simulink model "modules"  (R2017a)
settings: Solver=ode4  StartTime=0.0  StopTime=time_stop  FixedStep=time_step  RelTol=1e-3
values from neighbouring files (symbols this model uses):
  psi = state(3)    [PSVobstacleShip_class.m]    (also in PSVvessel_class.m = obj.eta(3); PsiReferenceModel_class.m = obj.desired_psi_vector; SBMPC_PSVvessel_class.m = obj.eta(3))
undefined symbols (not defined in the file or in its folder): beta, Delta_guidance, Delta_matrix, eta_initial, initial_desired_psi_vector, initial_desired_u_vector, initial_next_waypoint_indexes, initial_obstacle_ship_states, initial_obstacle_ship_states_dot, initial_reference_psi_vector, initial_reference_u_vector, initial_SBMPC_desired_psi_vector, initial_SBMPC_desired_u_vector, initial_SBMPC_next_waypoint_indexes, initial_SBMPC_obstacle_ship_states, initial_SBMPC_obstacle_ship_states_dot, initial_SBMPC_reference_psi_vector, initial_SBMPC_reference_u_vector, initial_SBMPC_x_d_psi_matrix, initial_SBMPC_x_d_u_matrix, initial_state, initial_x_d_psi_matrix, initial_x_d_u_matrix, K_sway, K_yaw, Kp_feedback_linearization, kp_heading, Nmax, nu_initial, num_obs_ship_waypoints, num_prediction_time_steps, number_of_control_behaviors, number_of_obstacle_ships, number_of_SBMPC_obstacle_ships, obs_speed_between_waypoints, obstacle_waypoint_matrix, Omega_matrix, own_ship_reference_psi_init, own_ship_reference_speed, Psi_init, radius_of_acceptance, SBMPC_obs_speed_between_waypoints, SBMPC_obstacle_waypoint_matrix, seconds_between_prediction, state_vector_init, T, T_k_surge, T_k_sway, T_k_yaw, T_s, T_waypoints, time_step, tsamp, U, U_init, V_init, waypoints_obstacle_ships, waypoints_own_ship, Xmax, Ymax
(part 4 of 5)

== matlab function modules/SBMPC obstacle ships/SBMPC using intentions /Calculate control behaviors/Compute hazard ==
  settings: updateMethod=DISCRETE  sampleTime=time_step
  data: obstacle_ships_u_input input size=[1 + number_of_obstacle_ships, num_prediction_time_steps]; obstacle_ships_v_input input size=[1 + number_of_obstacle_ships, num_prediction_time_steps]; obstacle_ships_psi_input input size=[1 + number_of_obstacle_ships, num_prediction_time_steps]; t_0 input; SBMPC_obstacles_own_ship_x_predicted input size=[number_of_SBMPC_obstacle_ships, num_prediction_time_steps, number_of_control_behaviors]; SBMPC_obstacles_own_ship_y_predicted input size=[number_of_SBMPC_obstacle_ships, num_prediction_time_steps, number_of_control_behaviors]; SBMPC_obstacles_own_ship_u_predicted input size=[number_of_SBMPC_obstacle_ships, num_prediction_time_steps, number_of_control_behaviors]; SBMPC_obstacles_own_ship_v_predicted input size=[number_of_SBMPC_obstacle_ships, num_prediction_time_steps, number_of_control_behaviors]; SBMPC_obstacles_own_ship_heading_predicted input size=[number_of_SBMPC_obstacle_ships, num_prediction_time_steps, number_of_control_behaviors]; CLOSE output size=[number_of_SBMPC_obstacle_ships, number_of_control_behaviors, total_number_of_obstacle_ships, num_prediction_time_steps]; d_0 output size=[number_of_SBMPC_obstacle_ships, number_of_control_behaviors, total_number_of_obstacle_ships, num_prediction_time_steps]; obstacle_ships_x_predicted_input input size=[1 + number_of_obstacle_ships, num_prediction_time_steps]; obstacle_ships_y_predicted_input input size=[1 + number_of_obstacle_ships, num_prediction_time_steps]; OVERTAKEN output size=[number_of_SBMPC_obstacle_ships, number_of_control_behaviors, total_number_of_obstacle_ships, num_prediction_time_steps]; STARBOARD output size=[number_of_SBMPC_obstacle_ships, number_of_control_behaviors, total_number_of_obstacle_ships, num_prediction_time_steps]; chosen_HEAD_ON_out output; CROSSED output size=[number_of_SBMPC_obstacle_ships, number_of_control_behaviors, total_number_of_obstacle_ships, num_prediction_time_steps]; mu output size=[number_of_SBMPC_obstacle_ships, number_of_control_behaviors, total_number_of_obstacle_ships, num_prediction_time_steps]; num_prediction_time_steps parameter; heading_angle_offset_commands parameter; propulsion_commands parameter; total_number_of_obstacle_ships parameter; seconds_between_prediction parameter; d_cl parameter; phi_head_on parameter; phi_crossed parameter; phi_overtaken parameter; phi_ahead parameter; K_coll parameter; C output size=[number_of_SBMPC_obstacle_ships, number_of_control_behaviors, total_number_of_obstacle_ships, num_prediction_time_steps]; R output size=[number_of_SBMPC_obstacle_ships, number_of_control_behaviors, total_number_of_obstacle_ships, num_prediction_time_steps]; q parameter; p parameter; d_safe parameter; k_boundary parameter; k_circle parameter; k_Pr parameter; k_psi_port parameter; k_psi_starboard parameter; Delta_Pr parameter; vessel_length parameter; circle_obstacle_parameters parameter; boundary_obstacles_parameters parameter; k_Delta_psi_port parameter; k_Delta_psi_starboard parameter; kappa parameter; f output size=[number_of_SBMPC_obstacle_ships,number_of_control_behaviors]; g output size=[number_of_SBMPC_obstacle_ships,number_of_control_behaviors]; hazard output size=[number_of_SBMPC_obstacle_ships,number_of_control_behaviors]; rad2deg parameter; num_boundary_obstacles parameter; num_circle_obstacles parameter; chosen_C_out output; chosen_FC_out output; chosen_R_out output; chosen_scaled_mu_out output; T_s parameter; chosen_Pr_out output; chosen_psi_ca_out output; C_worst output; R_worst output; scaled_mu_worst output; Pr_worst output; psi_ca_worst output; f_worst_out output; g_worst_out output; smallest_hazard_out output; largest_hazard_out output; f_out output; g_out output; r parameter; circle_safety_margin parameter; p_boundary parameter; p_circle parameter; q_circle parameter; q_boundary parameter; boundary_margin parameter; number_of_control_behaviors parameter; chosen_scenario_index_out output; number_of_SBMPC_obstacle_ships parameter; chosen_scenario_index_out_init parameter; data_out_init parameter; number_of_obstacle_ships parameter; L_FC parameter; k_FC parameter; L_C parameter
function [CLOSE, d_0, OVERTAKEN, STARBOARD, chosen_HEAD_ON_out, CROSSED,mu, C, R, f, g, hazard, chosen_C_out, chosen_FC_out, chosen_R_out, chosen_scaled_mu_out, chosen_Pr_out, chosen_psi_ca_out, C_worst, R_worst, scaled_mu_worst, Pr_worst, psi_ca_worst, f_worst_out, g_worst_out, smallest_hazard_out, largest_hazard_out, f_out, g_out, chosen_scenario_index_out]                         = computeTotalHazard(obstacle_ships_u_input, obstacle_ships_v_input, obstacle_ships_psi_input, t_0,SBMPC_obstacles_own_ship_x_predicted, SBMPC_obstacles_own_ship_y_predicted,SBMPC_obstacles_own_ship_u_predicted,SBMPC_obstacles_own_ship_v_predicted, SBMPC_obstacles_own_ship_heading_predicted, obstacle_ships_x_predicted_input, obstacle_ships_y_predicted_input, num_prediction_time_steps, heading_angle_offset_commands, propulsion_commands, total_number_of_obstacle_ships, seconds_between_prediction, d_cl,phi_head_on, phi_crossed, phi_overtaken,phi_ahead,K_coll, q, p, d_safe,k_boundary, k_circle, k_Pr, k_psi_port, k_psi_starboard, Delta_Pr, vessel_length, circle_obstacle_parameters, boundary_obstacles_parameters, k_Delta_psi_port, k_Delta_psi_starboard,kappa, rad2deg, num_boundary_obstacles, num_circle_obstacles, T_s, r, circle_safety_margin, p_boundary, p_circle, q_circle, q_boundary, boundary_margin, number_of_control_behaviors, number_of_SBMPC_obstacle_ships, chosen_scenario_index_out_init, data_out_init, number_of_obstacle_ships, L_FC, k_FC, L_C)     
    
    persistent chosen_C;
    persistent chosen_scenario_index;
    persistent chosen_R;
    persistent chosen_scaled_mu;
    persistent chosen_HEAD_ON;
    persistent chosen_FC;
    persistent chosen_Pr;
    persistent chosen_psi_ca;
    persistent chosen_Pr_worst;
    persistent chosen_psi_ca_worst;
    persistent f_worst;
    persistent g_worst;
    persistent f_chosen;
    persistent g_chosen;
    persistent smallest_hazard;
    persistent largest_hazard;
    persistent scenario_index_with_min_hazard;
    persistent scenario_index_with_max_hazard;
    
    if (isempty(chosen_C))
        chosen_C              = zeros(number_of_SBMPC_obstacle_ships,number_of_control_behaviors);%chosen_C_init;
        chosen_scenario_index = ones(1,number_of_SBMPC_obstacle_ships)*7;
        chosen_R              = zeros(number_of_SBMPC_obstacle_ships,number_of_control_behaviors);%chosen_R_init;
        chosen_scaled_mu      = zeros(number_of_SBMPC_obstacle_ships,number_of_control_behaviors);%chosen_scaled_mu_init; 
        chosen_FC             = zeros(number_of_SBMPC_obstacle_ships,number_of_control_behaviors);
        chosen_HEAD_ON        = zeros(number_of_SBMPC_obstacle_ships,number_of_control_behaviors);
        chosen_Pr             = ones(1, number_of_SBMPC_obstacle_ships);
        chosen_psi_ca         = data_out_init;
        chosen_Pr_worst       = data_out_init;
        chosen_psi_ca_worst   = data_out_init;
        f_worst               = data_out_init;
        g_worst               = data_out_init;
        f_chosen              = data_out_init;
        g_chosen              = data_out_init;
        smallest_hazard       = data_out_init;
        largest_hazard        = data_out_init;
        scenario_index_with_min_hazard = ones(1, number_of_SBMPC_obstacle_ships)*(-1);
        scenario_index_with_max_hazard = ones(1, number_of_SBMPC_obstacle_ships)*(-1);
        
    end
    
    chosen_scenario_index_out = chosen_scenario_index_out_init;

    CLOSE     = zeros(number_of_SBMPC_obstacle_ships, number_of_control_behaviors, total_number_of_obstacle_ships, num_prediction_time_steps);
    OVERTAKEN = zeros(number_of_SBMPC_obstacle_ships, number_of_control_behaviors, total_number_of_obstacle_ships, num_prediction_time_steps);
    STARBOARD = zeros(number_of_SBMPC_obstacle_ships, number_of_control_behaviors, total_number_of_obstacle_ships, num_prediction_time_steps);
    HEAD_ON   = zeros(number_of_SBMPC_obstacle_ships, number_of_control_behaviors, total_number_of_obstacle_ships, num_prediction_time_steps);
    CROSSED   = zeros(number_of_SBMPC_obstacle_ships, number_of_control_behaviors, total_number_of_obstacle_ships, num_prediction_time_steps);
    mu        = zeros(number_of_SBMPC_obstacle_ships, number_of_control_behaviors, total_number_of_obstacle_ships, num_prediction_time_steps);
    scaled_mu = zeros(number_of_SBMPC_obstacle_ships, number_of_control_behaviors, total_number_of_obstacle_ships, num_prediction_time_steps);
    d_0       = zeros(number_of_SBMPC_obstacle_ships, number_of_control_behaviors, total_number_of_obstacle_ships, num_prediction_time_steps);
    f         = zeros(number_of_SBMPC_obstacle_ships,number_of_control_behaviors);
    g         = zeros(number_of_SBMPC_obstacle_ships,number_of_control_behaviors);
    chosen_HEAD_ON_out   = data_out_init;
    chosen_C_out         = data_out_init;
    chosen_FC_out        = data_out_init;
    
    chosen_R_out         = data_out_init;
    chosen_scaled_mu_out =data_out_init;
    chosen_Pr_out        = data_out_init;
    chosen_psi_ca_out    = data_out_init;
    C_worst              = data_out_init;
    P_worst              = data_out_init;
    R_worst              = data_out_init;
    scaled_mu_worst      = data_out_init;
    Pr_worst             = data_out_init;
    psi_ca_worst         =data_out_init;
    f_worst_out          = data_out_init;
    g_worst_out          = data_out_init;
    smallest_hazard_out  = data_out_init;
    largest_hazard_out   = data_out_init;
    f_out                = data_out_init;
    g_out                = data_out_init;
    %R_vector_out         = zeros(number_of_control_behaviors, total_number_of_obstacle_ships, num_prediction_time_steps, number_of_SBMPC_obstacle_ships);
    %chosen_scenario_index_out  = zeros(1, number_of_SBMPC_obstacle_ships);
    %own_ship_u_predicted       = zeros(number_of_SBMPC_obstacle_ships, num_prediction_time_steps, number_of_control_behaviors);
    %own_ship_v_predicted       = zeros(num_prediction_time_steps, number_of_control_behaviors, number_of_SBMPC_obstacle_ships);
    %own_ship_heading_predicted = zeros(num_prediction_time_steps, number_of_control_behaviors, number_of_SBMPC_obstacle_ships);
    %own_ship_x_predicted       = zeros(num_prediction_time_steps, number_of_control_behaviors, number_of_SBMPC_obstacle_ships);
    %own_ship_y_predicted       = zeros(num_prediction_time_steps, number_of_control_behaviors, number_of_SBMPC_obstacle_ships);  
    
    obstacle_ships_u           = zeros(num_prediction_time_steps, total_number_of_obstacle_ships );
    obstacle_ships_v           = zeros(num_prediction_time_steps, total_number_of_obstacle_ships );
    obstacle_ships_psi         = zeros(num_prediction_time_steps, total_number_of_obstacle_ships );
    obstacle_ships_x_predicted = zeros(num_prediction_time_steps, total_number_of_obstacle_ships);
    obstacle_ships_y_predicted = zeros(num_prediction_time_steps, total_number_of_obstacle_ships);
    
    if (num_circle_obstacles > 0)
        g_circle_init  = zeros(number_of_control_behaviors, num_circle_obstacles, num_prediction_time_steps);
    else
        g_circle_init = 0;
    end    
    if (num_boundary_obstacles > 0)
        g_boundary_init = zeros(number_of_control_behaviors, num_boundary_obstacles, num_prediction_time_steps);
    else
        g_boundary_init = 0;
    end 
    g_circle  = g_circle_init;       %3D matrix. 1. dim = scneario, 2. dim = circle obstacle index, 3. dim = prediction horizon time step.
    g_boundary = g_boundary_init;    %3D matrix. 1. dim = scneario, 2. dim = circle obstacle index, 3. dim = prediction horizon time step.
    C = zeros(number_of_SBMPC_obstacle_ships, number_of_control_behaviors, total_number_of_obstacle_ships, num_prediction_time_steps);%C_init; %cost of collision. 3D matrix, 1. dim: scenario, 2. dim: obstacle, 3. dim: prediction horizon time step.
    R = zeros(number_of_SBMPC_obstacle_ships, number_of_control_behaviors, total_number_of_obstacle_ships, num_prediction_time_steps);%R_init; %Risk of collision. 3D matrix, 1. dim: scenario, 2. dim: obstacle, 3. dim: prediction horizon time step.
    hazard = zeros(number_of_SBMPC_obstacle_ships,number_of_control_behaviors); %hazard_init;
    FC     = zeros(number_of_SBMPC_obstacle_ships, number_of_control_behaviors, total_number_of_obstacle_ships, num_prediction_time_steps);%FC_init;   
    
    Pr_last = chosen_Pr;     %the Pr corresponding to the previously calculated lowest hazard.
    psi_ca_last = chosen_psi_ca;    
    if (t_0 == 0)
        Pr_last = ones(1, number_of_SBMPC_obstacle_ships);
        psi_ca_last = zeros(1, number_of_SBMPC_obstacle_ships);
    end
    prev_chosen_scenario_index = chosen_scenario_index;
    
    if (mod(t_0, seconds_between_prediction) == 0) %only compute every 10th second.
        
          for SBMPC_own_ship_index = 1:number_of_SBMPC_obstacle_ships
           %add SBMPC obstacle ships' data to obsatcle ship data for all sbmpc obstacle vessels except for SBMPC_own_ship_index.
           %obs data: x_predicted, y_predicted, psi, u, v, 
           %obs ship data from function "combine normal obs and own-ship obs ship data" contains own-ship module's vessel data as first element, then normal obs data, and sbmpc obstacle's data can be added at the end. 
           
           index_list = [1:number_of_SBMPC_obstacle_ships];
           SBMPC_obstacle_indexes = index_list(:,[1:(SBMPC_own_ship_index-1),(SBMPC_own_ship_index+1):end]);  %list of index values of all SBMPC obstacles EXCEPT for the SBMPC obstacle chosen to be the own-ship. 
           
           predicted_data_size = size(obstacle_ships_x_predicted_input);
           predicted_data_length = predicted_data_size(1);           
           
           obstacle_ships_u(:,1:predicted_data_length) = obstacle_ships_u_input';
           obstacle_ships_v(:,1:predicted_data_length) = obstacle_ships_v_input';
           obstacle_ships_psi(:,1:predicted_data_length) =obstacle_ships_psi_input';
           obstacle_ships_x_predicted(:,1:predicted_data_length) = obstacle_ships_x_predicted_input';
           obstacle_ships_y_predicted(:,1:predicted_data_length) = obstacle_ships_y_predicted_input';

           counter = 0;
           for index = 1:length(SBMPC_obstacle_indexes)
               counter = counter + 1;
               i = SBMPC_obstacle_indexes(index);
               obstacle_ships_u(:,predicted_data_length + counter)   = SBMPC_obstacles_own_ship_u_predicted(i,:,prev_chosen_scenario_index(i));
               obstacle_ships_v(:,predicted_data_length + counter)   = SBMPC_obstacles_own_ship_v_predicted(i,:,prev_chosen_scenario_index(i));
               obstacle_ships_psi(:,predicted_data_length + counter) = SBMPC_obstacles_own_ship_heading_predicted(i,:,prev_chosen_scenario_index(i));
               obstacle_ships_x_predicted(:, predicted_data_length + counter) =  SBMPC_obstacles_own_ship_x_predicted(i,:,prev_chosen_scenario_index(i)); %one row for each prediction time step and one column for each ship
               obstacle_ships_y_predicted(:, predicted_data_length + counter) =  SBMPC_obstacles_own_ship_y_predicted(i,:,prev_chosen_scenario_index(i));   
           end % end for    
           
           
           
           own_ship_u_predicted = reshape( SBMPC_obstacles_own_ship_u_predicted(SBMPC_own_ship_index,:,:) , [num_prediction_time_steps, number_of_control_behaviors]);
           own_ship_v_predicted = reshape( SBMPC_obstacles_own_ship_v_predicted(SBMPC_own_ship_index,:,:) , [num_prediction_time_steps, number_of_control_behaviors]);
           own_ship_heading_predicted = reshape( SBMPC_obstacles_own_ship_heading_predicted(SBMPC_own_ship_index,:,:) , [num_prediction_time_steps, number_of_control_behaviors]);
           own_ship_x_predicted = reshape( SBMPC_obstacles_own_ship_x_predicted(SBMPC_own_ship_index,:,:) , [num_prediction_time_steps, number_of_control_behaviors]);
           own_ship_y_predicted = reshape( SBMPC_obstacles_own_ship_y_predicted(SBMPC_own_ship_index,:,:) , [num_prediction_time_steps, number_of_control_behaviors]);
           
           
           
           scenario_index = 0;
           for Pr = propulsion_commands
               for psi_ca = heading_angle_offset_commands 
                   scenario_index = scenario_index + 1;                      
                   prediction_time = 0;
                   for t=1:num_prediction_time_steps   
                        prediction_time = t_0 + t*T_s;  
                        %Penalty for static obstacles   
                        if (num_circle_obstacles > 0)
                            circle_obs_counter = 0;
                            for circle_obstacle = circle_obstacle_parameters.'         %in each iteration, circle_obstacle is column vector with [radius; center_x; center_y]
                                circle_obs_counter = circle_obs_counter + 1;
                                radius    = circle_obstacle(1);
                                center_x  = circle_obstacle(2);
                                center_y  = circle_obstacle(3);
                                crossing_with_circle = SBMPC_isCollisionWithCircleObstacle(own_ship_x_predicted(t,scenario_index), own_ship_y_predicted(t,scenario_index), vessel_length, own_ship_heading_predicted(t,scenario_index), center_x, center_y, radius, circle_safety_margin);                       
                                vessel_bow_x = own_ship_x_predicted(t,scenario_index) + cos(own_ship_heading_predicted(t,scenario_index))*(vessel_length/2);
                                vessel_bow_y = own_ship_y_predicted(t,scenario_index) + sin(own_ship_heading_predicted(t,scenario_index))*(vessel_length/2);
                                distance_bow_to_circle_center = sqrt( (center_x - vessel_bow_x)^2 + (center_y - vessel_bow_y)^2 );
                                g_circle(scenario_index, circle_obs_counter, t) = (crossing_with_circle+1)*k_circle*(1/(prediction_time - t_0)^p_circle)*((radius+L_C)/ distance_bow_to_circle_center)^q_circle;%*(psi_ca*rad2deg)     * (1/distance_bow_to_circle_center)                   
                           end % end for circle obs
                        end % end if                        

                        if (num_boundary_obstacles > 0)
                            boundary_obs_counter = 0;
                            for boundary_obstacle = boundary_obstacles_parameters.'
                                boundary_obs_counter = boundary_obs_counter + 1;
                                boundary_start_x = boundary_obstacle(1);
                                boundary_start_y = boundary_obstacle(2);
                                boundary_end_x   = boundary_obstacle(3);
                                boundary_end_y   = boundary_obstacle(4);  
                                vessel_bow_x = own_ship_x_predicted(t,scenario_index) + cos(own_ship_heading_predicted(t,scenario_index))*(vessel_length/2);
                                vessel_bow_y = own_ship_y_predicted(t,scenario_index) + sin(own_ship_heading_predicted(t,scenario_index))*(vessel_length/2);
                                distance_bow_to_line = dist_from_bow_to_line( vessel_bow_x, vessel_bow_y, boundary_start_x, boundary_start_y, boundary_end_x, boundary_end_y ); % from http://paulbourke.net/geometry/pointlineplane/
                                crossing_with_boundary = SBMPC_isCollisionWithBoundaryObstacle(own_ship_x_predicted(t,scenario_index), own_ship_y_predicted(t,scenario_index), vessel_length, own_ship_heading_predicted(t,scenario_index), boundary_start_x, boundary_start_y, boundary_end_x, boundary_end_y);
                                g_boundary(scenario_index, boundary_obs_counter, t) = (crossing_with_boundary+1)*k_boundary*( 1 / (prediction_time - t_0)^p_boundary )*((boundary_margin)/(distance_bow_to_line))^q_boundary;  %from wiki https://en.wikipedia.org/wiki/Distance_from_a_point_to_a_line
                            end % end for boundary obs
                        end % end if
                        
                        for obstacle_ship_index = 1:total_number_of_obstacle_ships
                            obstacle_ship_speed = sqrt(obstacle_ships_u(t,obstacle_ship_index)^2 + obstacle_ships_v(t,obstacle_ship_index)^2);
                            own_ship_speed = sqrt(own_ship_u_predicted(t,scenario_index)^2 + own_ship_v_predicted(t,scenario_index)^2);
                            own_ship_u_NED = own_ship_speed*cos(own_ship_heading_predicted(t,scenario_index));
                            own_ship_v_NED = own_ship_speed*sin(own_ship_heading_predicted(t,scenario_index));
                            obstacle_ship_u_NED = obstacle_ship_speed*cos(obstacle_ships_psi(t,obstacle_ship_index));  
                            obstacle_ship_v_NED = obstacle_ship_speed*sin(obstacle_ships_psi(t,obstacle_ship_index));               
                            V_0 = [own_ship_u_NED,own_ship_v_NED];
                            V_i = [obstacle_ship_u_NED, obstacle_ship_v_NED];       

                            d_0(SBMPC_own_ship_index, scenario_index, obstacle_ship_index, t) = sqrt((own_ship_x_predicted(t,scenario_index) - obstacle_ships_x_predicted(t,obstacle_ship_index))^2 ...
                                                                            +  (own_ship_y_predicted(t,scenario_index) - obstacle_ships_y_predicted(t,obstacle_ship_index))^2); 


                            %%%% CLOSE

                            if (d_0(SBMPC_own_ship_index, scenario_index, obstacle_ship_index, t) <= d_cl(obstacle_ship_index))
                                CLOSE(SBMPC_own_ship_index, scenario_index, obstacle_ship_index, t) = 1;
                            else
                                CLOSE(SBMPC_own_ship_index, scenario_index, obstacle_ship_index, t) = 0;
                            end % end if

                            %%%% OVERTAKEN                  
                            %equation 5 in johansen
                            epsilon = 1;
                            if (CLOSE(SBMPC_own_ship_index, scenario_index, obstacle_ship_index, t) == 1 && obstacle_ship_speed > own_ship_speed + epsilon && dot(V_0, V_i) > cos(phi_overtaken)*norm(V_0)*norm(V_i))
                                OVERTAKEN(SBMPC_own_ship_index, scenario_index, obstacle_ship_index, t) = 1;
                            else
                                OVERTAKEN(SBMPC_own_ship_index, scenario_index, obstacle_ship_index, t) = 0;
                            end % end if

                            %%%% STARBOARD
                            L = [ obstacle_ships_x_predicted(t,obstacle_ship_index) - own_ship_x_predicted(t,scenario_index) , obstacle_ships_y_predicted(t,obstacle_ship_index) - own_ship_y_predicted(t,scenario_index) ];
                            L_unit_vector = L/norm(L);
                            L_angle = atan2(  (obstacle_ships_y_predicted(t,obstacle_ship_index) - own_ship_y_predicted(t,scenario_index)) , (obstacle_ships_x_predicted(t,obstacle_ship_index) - own_ship_x_predicted(t,scenario_index))  );

                            if (L_angle > own_ship_heading_predicted(t,scenario_index))
                                STARBOARD(SBMPC_own_ship_index, scenario_index, obstacle_ship_index, t) = 1;
                            else
                                STARBOARD(SBMPC_own_ship_index, scenario_index, obstacle_ship_index, t) = 0;
                            end
                            %rad2deg = 180/pi;
                            %L_angle_deg = L_angle*rad2deg;
                            %L_angle_deg_converted_to_positive =  mod((L_angle_deg + 360), 360);
                            %L_angle_mapped = L_angle_deg_converted_to_positive*deg2rad;  %map negative angles to positive angles.

                            %%%% HEAD_ON
                            head_on_condition = false;
                            if ( dot(V_0, V_i) < -cos(phi_head_on)*norm(V_0)*norm(V_i) && dot(V_0, L_unit_vector) > cos(phi_ahead)*norm(V_0) ) 
                                head_on_condition = true ; %equation 6-7 in johansen paper 
                            end% end if

                            if (CLOSE(SBMPC_own_ship_index, scenario_index, obstacle_ship_index, t) == 1 && norm(V_i) ~= 0 && head_on_condition == true )
                                HEAD_ON(SBMPC_own_ship_index, scenario_index, obstacle_ship_index, t) = 1;
                            else
                                HEAD_ON(SBMPC_own_ship_index, scenario_index, obstacle_ship_index, t) = 0;
                            end % end if

                            %%%% CROSSED                                              
                            if (CLOSE(SBMPC_own_ship_index, scenario_index, obstacle_ship_index, t) == 1 && dot(V_0, V_i) < cos(phi_crossed)*norm(V_0)*norm(V_i))
                                CROSSED(SBMPC_own_ship_index, scenario_index, obstacle_ship_index, t) = 1;
                            else
                                CROSSED(SBMPC_own_ship_index, scenario_index, obstacle_ship_index, t) = 0;
                            end % end if

                            %%%% RULE14    
                            if (CLOSE(SBMPC_own_ship_index, scenario_index, obstacle_ship_index, t) == 1 && STARBOARD(SBMPC_own_ship_index, scenario_index, obstacle_ship_index, t) == 1 && HEAD_ON(SBMPC_own_ship_index, scenario_index, obstacle_ship_index, t) == 1 )
                                RULE14 = true;
                            else
                                RULE14 = false;
                            end % end if

                            %%%% RULE15   
                            if (CLOSE(SBMPC_own_ship_index, scenario_index, obstacle_ship_index, t) == 1 && STARBOARD(SBMPC_own_ship_index, scenario_index, obstacle_ship_index, t) == 1 && CROSSED(SBMPC_own_ship_index, scenario_index, obstacle_ship_index, t) == 1 && OVERTAKEN(SBMPC_own_ship_index, scenario_index, obstacle_ship_index, t) == 0 )
                                RULE15 = true;
                            else
                                 RULE15 = false;
                            end % end if

                            %%%% mu
                            if (RULE14 || RULE15)
                                mu(SBMPC_own_ship_index, scenario_index, obstacle_ship_index, t) = 1;
                            else
                                mu(SBMPC_own_ship_index, scenario_index, obstacle_ship_index, t) = 0;
                            end % end if                         
                            scaled_mu(SBMPC_own_ship_index, scenario_index, obstacle_ship_index, t) = kappa(obstacle_ship_index)*mu(SBMPC_own_ship_index, scenario_index, obstacle_ship_index, t);



                            %%%% Cost of collision
                            C(SBMPC_own_ship_index, scenario_index, obstacle_ship_index, t) = K_coll(obstacle_ship_index)*norm(V_0 - V_i)^2;

                            
                            
                            %%%% Risk of collision                       
                            if (d_0(SBMPC_own_ship_index, scenario_index, obstacle_ship_index, t) <= L_FC)
                                FC(SBMPC_own_ship_index, scenario_index, obstacle_ship_index, t) = 1;
                            else
                                FC(SBMPC_own_ship_index, scenario_index, obstacle_ship_index, t) = 0;
                            end % end if
                            
                            if (d_0(SBMPC_own_ship_index, scenario_index, obstacle_ship_index, t) <= d_safe(obstacle_ship_index) && d_0(SBMPC_own_ship_index, scenario_index, obstacle_ship_index, t) >= 20)                          
                                R(SBMPC_own_ship_index, scenario_index, obstacle_ship_index, t)  = (1 / (abs(prediction_time - t_0)^p))*( r*( d_safe(obstacle_ship_index) / d_0(SBMPC_own_ship_index, scenario_index, obstacle_ship_index, t) )^q + k_FC*FC(SBMPC_own_ship_index, scenario_index, obstacle_ship_index, t)   ) ;
                                if ( R(SBMPC_own_ship_index, scenario_index, obstacle_ship_index, t) >= 20000)
                                    R(SBMPC_own_ship_index, scenario_index, obstacle_ship_index, t) = 20000;  %saturate
                                end
                            else
                                R(SBMPC_own_ship_index, scenario_index, obstacle_ship_index, t) = 0;
                            end % end if        

                        end % end for - num obs ships        
                   end % end for t
               end % end for psi_ca
            end % end for Pr
           
            scenario_index = 0;
            for Pr = propulsion_commands
                for psi_ca = heading_angle_offset_commands 
                    scenario_index = scenario_index + 1;
                    sum_matrix = C(SBMPC_own_ship_index,scenario_index,:,:).*R(SBMPC_own_ship_index, scenario_index,:,:) + scaled_mu(SBMPC_own_ship_index, scenario_index,:,:) ;   
                    sum_matrix = reshape(sum_matrix, total_number_of_obstacle_ships, num_prediction_time_steps);
                    [best_value,idx] = max(sum_matrix(:));
                    [best_obstacle_ship_index,best_timestep] = ind2sub(size(sum_matrix),idx);                          

                    if ( psi_ca < 0)
                        k_psi = k_psi_port;  
                        Delta_psi = k_Delta_psi_port*(abs(psi_ca*rad2deg - psi_ca_last(SBMPC_own_ship_index)*rad2deg));
                    else
                        k_psi = k_psi_starboard;
                        Delta_psi = k_Delta_psi_starboard*(abs(psi_ca*rad2deg - psi_ca_last(SBMPC_own_ship_index)*rad2deg));
                    end % end if                

                    f(SBMPC_own_ship_index, scenario_index) = k_Pr*(1-Pr) + k_psi*(abs(psi_ca*rad2deg)) + Delta_Pr*abs(Pr - Pr_last(SBMPC_own_ship_index)) + Delta_psi ;                                 

                    g_circle_scenario = 0;
                    if (num_circle_obstacles > 0)
                        g_circle_scenario_values = g_circle(scenario_index, :, :);
                        g_circle_scenario = max(g_circle_scenario_values(:));
                    end % end if                
                    g_boundary_scenario = 0;
                    if (num_boundary_obstacles > 0)
                        g_boundary_scenario_values = g_boundary(scenario_index, :, :);
                        g_boundary_scenario = max(g_boundary_scenario_values(:));
                    end % end if                
                    g(SBMPC_own_ship_index, scenario_index) = g_circle_scenario + g_boundary_scenario;

                    hazard(SBMPC_own_ship_index, scenario_index) = best_value + f(SBMPC_own_ship_index, scenario_index) + g(SBMPC_own_ship_index, scenario_index);

                    %The C, R and K*µ corresponding to the values used to find hazard H for scenario k.
                    chosen_C(SBMPC_own_ship_index, scenario_index) = C(SBMPC_own_ship_index,scenario_index,best_obstacle_ship_index,best_timestep);  %the C value used to compute hazard in scenario number "scenario_index"
                    chosen_R(SBMPC_own_ship_index, scenario_index) = R(SBMPC_own_ship_index,scenario_index,best_obstacle_ship_index,best_timestep);

                    chosen_scaled_mu(SBMPC_own_ship_index, scenario_index) = scaled_mu(SBMPC_own_ship_index, scenario_index,best_obstacle_ship_index,best_timestep);  
                    chosen_FC(SBMPC_own_ship_index, scenario_index)     = FC(SBMPC_own_ship_index, scenario_index,best_obstacle_ship_index,best_timestep)*k_FC;
                    assert (best_value == chosen_C(SBMPC_own_ship_index, scenario_index)*chosen_R(SBMPC_own_ship_index, scenario_index) + chosen_scaled_mu(SBMPC_own_ship_index, scenario_index) );                                           
                end % end for
            end % end for
            
            [min_hazard, scenario_index_with_min_hazard] = min(hazard(SBMPC_own_ship_index,:));
            [max_hazard, scenario_index_with_max_hazard] = max(hazard(SBMPC_own_ship_index,:));  
            smallest_hazard(SBMPC_own_ship_index) = min_hazard;
            largest_hazard(SBMPC_own_ship_index) = max_hazard;

            %h_min = hazard(SBMPC_own_ship_index,scenario_index_with_min_hazard);
            %h_max = hazard(SBMPC_own_ship_index,scenario_index_with_max_hazard);
            %assert(min_hazard == hazard(SBMPC_own_ship_index,scenario_index_with_min_hazard));
            %assert(max_hazard == h_max);

            f_chosen(SBMPC_own_ship_index) = f(SBMPC_own_ship_index, scenario_index_with_min_hazard);
            g_chosen(SBMPC_own_ship_index) = g(SBMPC_own_ship_index, scenario_index_with_min_hazard);
            f_worst(SBMPC_own_ship_index)  = f(SBMPC_own_ship_index, scenario_index_with_max_hazard);
            g_worst(SBMPC_own_ship_index)  = g(SBMPC_own_ship_index, scenario_index_with_max_hazard); 

            scenario_index = 0;
            for Pr = propulsion_commands
                for psi_ca = heading_angle_offset_commands
                    scenario_index = scenario_index +1;
                    if (scenario_index == scenario_index_with_min_hazard)
                        chosen_Pr(SBMPC_own_ship_index) = Pr;
                        chosen_psi_ca(SBMPC_own_ship_index) = psi_ca; 
                        chosen_scenario_index(SBMPC_own_ship_index) = scenario_index;
                    elseif (scenario_index == scenario_index_with_max_hazard)
                        chosen_Pr_worst(SBMPC_own_ship_index) = Pr;
                        chosen_psi_ca_worst(SBMPC_own_ship_index) = psi_ca;                   
                    end % end if
                end % end for
            end % end for               
         end % end for sbmpc obstacles                  
     end % end if
    
     
    for i = 1:number_of_SBMPC_obstacle_ships
        chosen_C_out(i) = chosen_C(i);
        chosen_scenario_index_out(i) = chosen_scenario_index(i);
        chosen_FC_out(i) = chosen_FC(i);
        chosen_HEAD_ON_out(i) = chosen_HEAD_ON(i);
        C_worst(i) = chosen_C(i);
        chosen_R_out(i) = chosen_R(i);
        R_worst(i) = chosen_R(i);
        chosen_scaled_mu_out(i) = chosen_scaled_mu(i);
        scaled_mu_worst(i) = chosen_scaled_mu(i);
        chosen_Pr_out(i) = chosen_Pr(i);
        Pr_worst(i) = chosen_Pr_worst(i);
        chosen_psi_ca_out(i) = chosen_psi_ca(i);
        psi_ca_worst(i) = chosen_psi_ca_worst(i);
        f_worst_out(i) = f_worst(i);
        g_worst_out(i) = g_worst(i);
        %R_vector_out(i) = R(SBMPC_own_ship_index,:, :, :);

        f_out(i) = f_chosen(i);
        g_out(i) = g_chosen(i);
        smallest_hazard_out(i) = smallest_hazard(i);
        largest_hazard_out(i) =  largest_hazard(i);   
    end
    
     
    

 end % end function

== matlab function modules/Own-ship/SBMPC /Predict obstacle trajectories/Normal obstacle ships trajectories prediction/Normal obstacle ships trajectories prediction ==
  settings: updateMethod=DISCRETE  sampleTime=time_step
  data: obstacle_ships_headings input; obstacle_ships_x_predicted output size=[num_prediction_time_steps, number_of_obstacle_ships]; obstacle_ships_y_predicted output size=[num_prediction_time_steps, number_of_obstacle_ships]; obstacle_ships_next_waypoint_index_vector input; obstacle_ships_initial_positions input; obstacle_ships_u input; obstacle_ships_v input; T_s parameter; t_0 input; number_of_obstacle_ships parameter; seconds_between_prediction parameter; num_prediction_time_steps parameter; obstacle_ships_u_predicted output size=[num_prediction_time_steps, number_of_obstacle_ships]; obstacle_ships_v_predicted output size=[num_prediction_time_steps, number_of_obstacle_ships]; obstacle_ships_psi_predicted output size=[num_prediction_time_steps, number_of_obstacle_ships]
function [obstacle_ships_x_predicted,obstacle_ships_y_predicted, obstacle_ships_u_predicted, obstacle_ships_v_predicted, obstacle_ships_psi_predicted] = normalObstacleShipsTrajectoryPrediction(obstacle_ships_headings, obstacle_ships_next_waypoint_index_vector, obstacle_ships_initial_positions, obstacle_ships_u, obstacle_ships_v, T_s, t_0, number_of_obstacle_ships, seconds_between_prediction, num_prediction_time_steps)
     deg2rad = pi/180;
     rad2deg = 180/pi;
     obstacle_ships_x_predicted = zeros( num_prediction_time_steps, number_of_obstacle_ships);   % obstacle_ships_x_predicted_init;  %%each row is a point in time, each column is an obstacle
     obstacle_ships_y_predicted = zeros( num_prediction_time_steps, number_of_obstacle_ships);   %obstacle_ships_y_predicted_init;  %%each row is a point in time, each column is an obstacle    
     obstacle_ships_u_predicted = zeros( num_prediction_time_steps, number_of_obstacle_ships);
     obstacle_ships_v_predicted = zeros( num_prediction_time_steps, number_of_obstacle_ships);
     obstacle_ships_psi_predicted = zeros( num_prediction_time_steps, number_of_obstacle_ships);
     if (mod(t_0, seconds_between_prediction) == 0)                 %Only do calculation every "seconds_between_prediction" second.
         for obstacle_ship_index = 1:number_of_obstacle_ships
             obstacle_ships_x_predicted(1, obstacle_ship_index) = obstacle_ships_initial_positions(obstacle_ship_index, 1);
             obstacle_ships_y_predicted(1, obstacle_ship_index) = obstacle_ships_initial_positions(obstacle_ship_index, 2);
             obstacle_ships_u_predicted(1, obstacle_ship_index) =obstacle_ships_u(obstacle_ship_index);
             obstacle_ships_v_predicted(1, obstacle_ship_index) = obstacle_ships_v(obstacle_ship_index);
             obstacle_ships_psi_predicted(1, obstacle_ship_index) = obstacle_ships_headings(obstacle_ship_index);
             for i = 2:num_prediction_time_steps
                obstacle_ship_speed = sqrt(obstacle_ships_u(obstacle_ship_index)^2 + obstacle_ships_v(obstacle_ship_index)^2);
                obstacle_ships_u_predicted(i,obstacle_ship_index) = obstacle_ships_u(obstacle_ship_index); %assume same speed for entire prediction horizon
                obstacle_ships_v_predicted(i,obstacle_ship_index) = obstacle_ships_v(obstacle_ship_index);
                obstacle_ships_psi_predicted(i, obstacle_ship_index) = obstacle_ships_headings(obstacle_ship_index);
                obstacle_ships_x_predicted(i,obstacle_ship_index) = obstacle_ships_x_predicted(i-1,obstacle_ship_index) + obstacle_ship_speed*cos(obstacle_ships_headings(obstacle_ship_index))*(T_s);   
                obstacle_ships_y_predicted(i,obstacle_ship_index) = obstacle_ships_y_predicted(i-1,obstacle_ship_index) + obstacle_ship_speed*sin(obstacle_ships_headings(obstacle_ship_index))*(T_s);
             end
             
         end % end for
     end % end if

end

== matlab function modules/Own-ship/guidance/waypoint guidance ==
  data: waypoints input; reference_psi output; vessel_position input; time_step parameter; beta parameter; Delta_guidance parameter; radius_of_acceptance parameter; next_waypoint_index output; own_ship_reference_psi_init parameter
function [reference_psi,next_waypoint_index]  = waypoint_guidance(waypoints, vessel_position, time_step, beta, Delta_guidance, radius_of_acceptance, own_ship_reference_psi_init)
    persistent waypointGuidanceObject;
    
    if (isempty(waypointGuidanceObject))
        waypointGuidanceObject = waypointGuidance_class(own_ship_reference_psi_init, waypoints, vessel_position, Delta_guidance, beta, time_step, radius_of_acceptance);
    end
    
    waypointGuidanceObject = waypointGuidanceObject.updateVesselPosition(vessel_position);
    waypointGuidanceObject = waypointGuidanceObject.updateCurrentWaypoint();
    [waypointGuidanceObject, reference_psi] = waypointGuidanceObject.getReferencePsi();    
    next_waypoint_index = waypointGuidanceObject.getNextwaypointIndex();
end

== matlab function modules/Own-ship/reference model nu/MATLAB Function ==
  data: reference_u input; nu_initial parameter; time_step parameter; x_d_new output; Delta_matrix parameter; Omega_matrix parameter
function x_d_new = ReferenceModelForSpeed(reference_u, nu_initial, time_step, Delta_matrix, Omega_matrix)    

persistent x_d %[nu; nu_dot] = [u,v,r, u_dot, v_dot, r_dot]

if isempty(x_d)
    x_d = [nu_initial;0;0;0];
end

x_d = speedReferenceModel(x_d, reference_u, time_step, Delta_matrix, Omega_matrix);
x_d_new = x_d;
end

== matlab function modules/SBMPC obstacle ships/SBMPC Obstacle vessels ==
  data: desired_psi_vector input; desired_u_vector input; SBMPC_obstacle_ships_state_matrix output; X output; Y output; Psi output; U output; V output; R output; SBMPC_obs_nu output; Nmax parameter; Ymax parameter; Xmax parameter; kp_heading parameter; Kp_feedback_linearization parameter; initial_SBMPC_obstacle_ship_states parameter; time_step parameter; initial_SBMPC_obstacle_ship_states_dot parameter; number_of_SBMPC_obstacle_ships parameter; K_sway parameter; K_yaw parameter; T_k_yaw parameter; T_k_sway parameter; T_k_surge parameter; Pr input; Psi_ca input; SBMPC_obs_eta output
function [SBMPC_obstacle_ships_state_matrix, X, Y, Psi, U, V, R, SBMPC_obs_nu, SBMPC_obs_eta] = SBMPCobstacleVessels(desired_psi_vector, desired_u_vector, Nmax, Ymax, Xmax, kp_heading, Kp_feedback_linearization, initial_SBMPC_obstacle_ship_states, time_step, initial_SBMPC_obstacle_ship_states_dot, number_of_SBMPC_obstacle_ships, K_sway, K_yaw,  T_k_yaw, T_k_sway, T_k_surge, Pr, Psi_ca)
    persistent obstacle_ships
    
    if (isempty(obstacle_ships))
        psvParameters = coder.load('PSVparameters');
        psvModelParameters = psvParameters.model_config;
        obstacle_ships = obstacleShips_class(number_of_SBMPC_obstacle_ships, initial_SBMPC_obstacle_ship_states, initial_SBMPC_obstacle_ship_states_dot, desired_psi_vector, desired_u_vector, time_step, psvModelParameters, Kp_feedback_linearization, kp_heading, Xmax, Ymax, Nmax, K_sway, K_yaw, T_k_surge, T_k_sway, T_k_yaw);
    end
    
    desired_psi_vector = desired_psi_vector + Psi_ca;
    desired_u_vector = desired_u_vector.*Pr;  %desired u is a row vector

    
    
    obstacle_ships = obstacle_ships.updateDesiredSpeedVector(desired_u_vector);
    obstacle_ships = obstacle_ships.updateDesiredPsiVector(desired_psi_vector);    
    obstacle_ships = obstacle_ships.updateObstacleShipsStates();
    
    %each column i in the obstacleShipsStateMatrix is the state [x,y,psi,u,v,r] for obstacle ship number i
    SBMPC_obstacle_ships_state_matrix = obstacle_ships.getObstacleShipsStateMatrix(); 

    %column vectors with states. Each element/column r is value for obstacle ship number r
    X = SBMPC_obstacle_ships_state_matrix(1,:);
    Y = SBMPC_obstacle_ships_state_matrix(2,:);
    Psi = SBMPC_obstacle_ships_state_matrix(3,:);
    U = SBMPC_obstacle_ships_state_matrix(4,:);
    V = SBMPC_obstacle_ships_state_matrix(5,:);
    R = SBMPC_obstacle_ships_state_matrix(6,:);   
    SBMPC_obs_eta = [X', Y', Psi'];  %each row i contains [x,y,psi] for obstacle ship i.
    SBMPC_obs_nu  = [U', V', R'];
end
